simulink model "TransferFunction"  (R2019a)
settings: Solver=VariableStepAuto  StartTime=0.0  StopTime=10.0  MaxStep=1 / 100  RelTol=1e-3
settings Model: Creator=Ali Mohamed  LastModifiedBy=Ali Mohamed

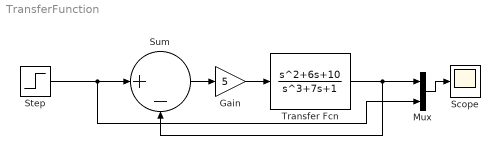
== system TransferFunction ==
  Gain : Gain  Gain=5
  Mux : Mux  Inputs=2
  Scope : Scope
  Step : Step  SampleTime=0
  Sum : Sum  Inputs=|+-
  Transfer Fcn : TransferFcn  Numerator=[1 6 10]  Denominator=[1 0 7 1]
  wires:
  Sum/1 -> Gain/1
  Transfer Fcn/1 -> Mux/1, Sum/2
  Mux/1 -> Scope/1
  Gain/1 -> Transfer Fcn/1
  Step/1 -> Mux/2, Sum/1
